simulink model "model3_image_qpsk_ofdm_awgn"  (R2025b)
settings: Solver=FixedStepDiscrete  StartTime=0.0  StopTime=1023  RelTol=1e-3
libraries: commofdm x2, commdigbbndpm3 x2, commchan3 x1
settings Model: Creator=Naren  LastModifiedBy=Naren

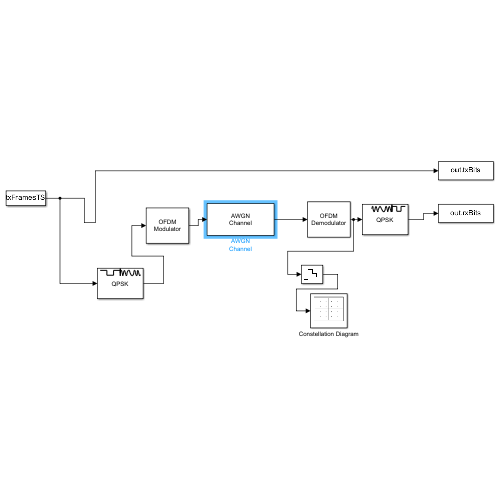
[thumbnail: Simulink's stored preview of the top-level diagram]
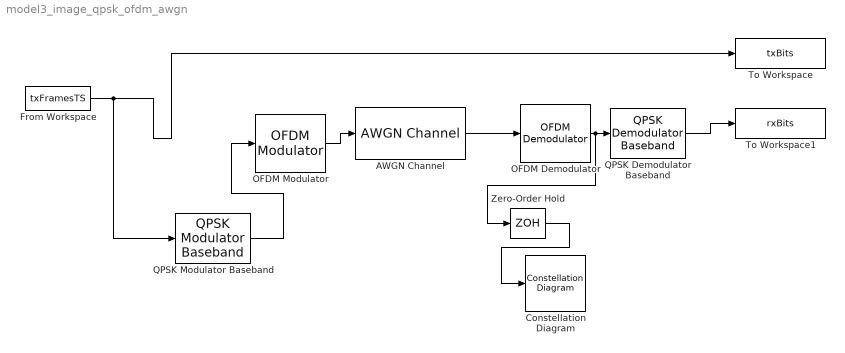
== system model3_image_qpsk_ofdm_awgn ==
  AWGN Channel : commchan3/AWGN Channel  LegacyMode=off  NoiseMethod="Signal to noise ratio  (SNR)"  noiseMode="Signal to noise ratio  (SNR)"  EbNo=10  EsNo=10  SNR=40  BitsPerSymbol=1  SignalPower=1  SpecifySymbolPeriod=off  SamplesPerSymbol=1  SymbolPeriod=1  VarianceSource=Parameter  Variance=1  RandomStream=Global stream  Seed=67  SimulateUsing=Code generation
  Constellation Diagram : ConstellationDiagram  WindowPosition=[660.000000,240.000000,600.000000,600.000000,]  ScopeFrameLocation=window  ShowLegend=on
  From Workspace : FromWorkspace  VariableName=txFramesTS
  OFDM Demodulator : commofdm/OFDM Demodulator  StatePerturbationForJacobian=1.0e-05  FFTLength=64  NumGuardBandCarriers=[7; 8]  RemoveDCCarrier=on  PilotOutputPort=off  PilotCarrierIndices=[12; 26; 40; 54]  CyclicPrefixLength=16  OversamplingFactor=1  NumSymbols=1  NumReceiveAntennas=1  SimulateUsing=Interpreted execution
  OFDM Modulator : commofdm/OFDM Modulator  StatePerturbationForJacobian=1.0e-05  FFTLength=64  NumGuardBandCarriers=[7; 8]  InsertDCNull=on  PilotInputPort=off  PilotCarrierIndices=[12; 26; 40; 54]  CyclicPrefixLength=16  Windowing=off  WindowLength=1  OversamplingFactor=1  NumSymbols=1  NumTransmitAntennas=1  SimulateUsing=Interpreted execution
  QPSK Demodulator Baseband : commdigbbndpm3/QPSK Demodulator Baseband  OutType=Bit  DecType=Hard decision  VarSource=Dialog  Variance=1  Dec=Gray  Ph=pi/4  outDtype1=Inherit via internal rule  outDtype2=Inherit via internal rule  derotateFactorWordLen=16  derotateFactorDataTypeStr=Inherit: Same word length as input  derotateFactorLastDataTypeStr=Inherit: Same word length as input
  QPSK Modulator Baseband : commdigbbndpm3/QPSK Modulator Baseband  InType=Bit  Enc=Gray  Ph=pi/4  outDtype=double  outWordLen=16  outUDDataType=sfix(16)  outFracLenMode=Best precision  outFracLen=15  outDataTypeStr=double  outLastDataTypeStr=double
  To Workspace : ToWorkspace  VariableName=txBits  SampleTime=-1
  To Workspace1 : ToWorkspace  VariableName=rxBits  SampleTime=-1
  Zero-Order Hold : ZeroOrderHold
  wires:
  AWGN Channel/1 -> OFDM Demodulator/1
  QPSK Demodulator Baseband/1 -> To Workspace1/1
  QPSK Modulator Baseband/1 -> OFDM Modulator/1
  OFDM Modulator/1 -> AWGN Channel/1
  OFDM Demodulator/1 -> Zero-Order Hold/1, QPSK Demodulator Baseband/1
  From Workspace/1 -> QPSK Modulator Baseband/1, To Workspace/1
  Zero-Order Hold/1 -> Constellation Diagram/1
